simulink model "SupervisorFSM_TX"  (R2023b)
settings: Solver=FixedStepDiscrete  StartTime=0.0  StopTime=10.0  FixedStep=Ts_SupervisorFSM_TX  RelTol=1e-3  EnableMultiTasking=on
libraries: simulink x2
settings Model: DataDictionary=EmbeddedBoardDD.sldd  Creator=vvasco  LastModifiedBy=upattacini
settings SolverCC: AllowMultiTaskInputOutput=on  AlgebraicLoopSolver=TrustRegion  AutoInsertRateTranBlk=on  InsertRTBMode=Never (minimum delay)
settings DataIOCC: LimitDataPoints=on  SaveOutput=off  SignalLogging=off  DSMLogging=off  SaveTime=off  ReturnWorkspaceOutputs=off
settings OptimizationCC: DefaultParameterBehavior=Inlined  DefaultUnderspecifiedDataType=single  StrengthReduction=on  PassReuseOutputArgsAs=Individual arguments  ZeroExternalMemoryAtStartup=off  ZeroInternalMemoryAtStartup=off  OptimizeBlockOrder=speed  OptimizationPriority=Speed  OptimizationCustomize=off  MultiThreadedLoops=on  EfficientTunableParamExpr=on
settings DebuggingCC: ParameterPrecisionLossMsg=none  UnconnectedInputMsg=warning  UnconnectedOutputMsg=warning  UnconnectedLineMsg=warning  AllowSymbolicDim=off  SFUnexpectedBacktrackingDiag=warning  SFNoUnconditionalDefaultTransitionDiag=warning  SFExecutionAtInitializationDiag=none  ArithmeticOperatorsInVariantConditions=warning
settings HardwareCC: ProdBitPerPointer=32  ProdBitPerSizeT=32  ProdBitPerPtrDiffT=32  ProdLargestAtomicInteger=Long  ProdLargestAtomicFloat=Double  ProdWordSize=32  ProdHWDeviceType=ARM Compatible->ARM Cortex-M
settings ModelReferenceCC: UpdateModelReferenceTargets=Force  EnableRefExpFcnMdlSchedulingChecks=on  ModelReferenceNumInstancesAllowed=Single
settings SFSimCC: SimUseLocalCustomCode=off  MATLABDynamicMemAlloc=off  CustomCodeUndefinedFunction=UseInterfaceOnly
settings RTWCC: Description=Embedded Coder  SystemTargetFile=ert.tlc  GenCodeOnly=on  PackageGeneratedCodeAndArtifacts=on  PackageName=SupervisorFSM_TX  TemplateMakefile=ert_default_tmf  GenerateReport=on  RTWUseLocalCustomCode=off  LaunchReport=on  TargetLang=C++  GenerateCodeReplacementReport=on  DLArmComputeVersion=19.05
settings CodeAppCC: ForceParamTrailComments=on  IgnoreCustomStorageClasses=off  MaxIdLength=60  OperatorAnnotations=on  SimulinkDataObjDesc=on  SFDataObjDesc=on  InsertBlockDesc=on
settings ERTTargetCC: TargetLangStandard=C++03 (ISO)  CodeReplacementLibrary=ARM Cortex-M,iCubTech  GenerateSampleERTMain=on  SupportVariableSizeSignals=on  InlinedParameterPlacement=NonHierarchical  RootIOFormat=Structure reference  ERTCustomFileTemplate=example_file_process.tlc
settings ConfigComp: CovMetricSettings=dw  CovSaveCumulativeToWorkspaceVar=on  CovSaveSingleToWorkspaceVar=on  CovExternalEMLEnable=off

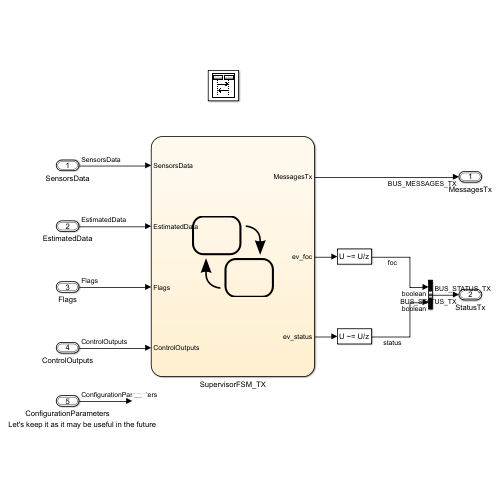
[thumbnail: Simulink's stored preview of the top-level diagram]
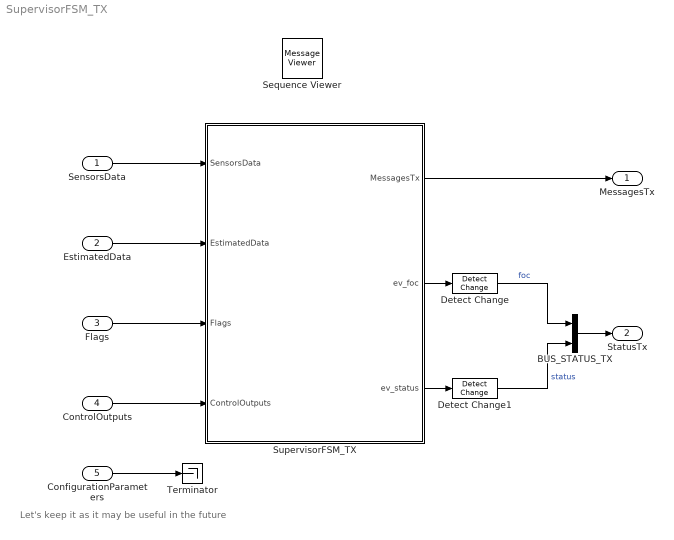
== system SupervisorFSM_TX ==
  note: Let's keep it as it may be useful in the future
  SensorsData : Inport  OutDataTypeStr=Bus: SensorsData  BusOutputAsStruct=on
  EstimatedData : Inport  Port=2  OutDataTypeStr=Bus: EstimatedData  BusOutputAsStruct=on
  Flags : Inport  Port=3  OutDataTypeStr=Bus: Flags  BusOutputAsStruct=on
  ControlOutputs : Inport  Port=4  OutDataTypeStr=Bus: ControlOutputs  BusOutputAsStruct=on
  ConfigurationParameters : Inport  Port=5  OutDataTypeStr=Bus: ConfigurationParameters  BusOutputAsStruct=on
  BUS_STATUS_TX : BusCreator  Inputs=2  OutDataTypeStr=Bus: BUS_STATUS_TX  NonVirtualBus=on
      settings: InheritFromInputs=off
  Detect Change : simulink/Logic and Bit Operations/Detect Change  vinit=false  OutDataTypeStr=boolean
  Detect Change1 : simulink/Logic and Bit Operations/Detect Change  vinit=false  OutDataTypeStr=boolean
  Sequence Viewer : MessageViewer  History=1000  SavedRootId=#
  SupervisorFSM_TX : Stateflow chart  TreatAsAtomicUnit=on
  Terminator : Terminator
  MessagesTx : Outport  OutDataTypeStr=Bus: BUS_MESSAGES_TX  BusOutputAsStruct=on
  StatusTx : Outport  Port=2  OutDataTypeStr=Bus: BUS_STATUS_TX  BusOutputAsStruct=on
  wires:
  SupervisorFSM_TX/1(MessagesTx) -> MessagesTx/1
  SensorsData/1 -> SupervisorFSM_TX/1(SensorsData)
  Flags/1 -> SupervisorFSM_TX/3(Flags)
  BUS_STATUS_TX/1 -> StatusTx/1
  EstimatedData/1 -> SupervisorFSM_TX/2(EstimatedData)
  ControlOutputs/1 -> SupervisorFSM_TX/4(ControlOutputs)
  SupervisorFSM_TX/2(ev_foc) -> Detect Change/1
  Detect Change/1 -> BUS_STATUS_TX/1  "foc"
  SupervisorFSM_TX/3(ev_status) -> Detect Change1/1
  Detect Change1/1 -> BUS_STATUS_TX/2  "status"
  ConfigurationParameters/1 -> Terminator/1

== stateflow chart SupervisorFSM_TX/SupervisorFSM_TX ==
  state MSG_FOC_HANDLER [parallel]
    settings: executionOrder=1
    state Home
    (default) -> MSG_FOC_HANDLER.Home
    MSG_FOC_HANDLER.Home -> MSG_FOC_HANDLER.Home : [Flags.enable_sending_msg_status]
        | {MessagesTx.foc.current = EstimatedData.Iq_filtered.current;
        | MessagesTx.foc.velocity = EstimatedData.jointvelocities.velocity;
        | MessagesTx.foc.position = SensorsData.jointpositions.position;
        | send(ev_foc);}
  state MSG_STATUS_HANDLER [parallel]
    settings: executionOrder=2
    state Home
    (default) -> MSG_STATUS_HANDLER.Home
    MSG_STATUS_HANDLER.Home -> MSG_STATUS_HANDLER.Home : [Flags.enable_sending_msg_status]
        | {MessagesTx.status.control_mode = convert(Flags.control_mode);
        | MessagesTx.status.pwm_fbk = ControlOutputs.Vq;
        | MessagesTx.status.flags.ExternalFaultAsserted = Flags.fault_button;
        | MessagesTx.status.flags.OverCurrentFailure = Flags.overcurrent;
        | send(ev_status);}
  data: mccontrolmode function_output Enum: MCControlModes size=1; controlmode function_input Enum: ControlModes size=1; MessagesTx output Bus: BUS_MESSAGES_TX; SensorsData input Bus: SensorsData; EstimatedData input Bus: EstimatedData; Flags input Bus: Flags; ControlOutputs input Bus: ControlOutputs
  events: ev_foc output EITHER_EDGE_EVENT; ev_status output EITHER_EDGE_EVENT
  function mccontrolmode = convert(controlmode):
    | function mccontrolmode = convert(controlmode)
    | 
    | if controlmode == ControlModes.Idle
    |     mccontrolmode = MCControlModes.Idle;
    | elseif controlmode == ControlModes.Current
    |     mccontrolmode = MCControlModes.Current;
    | elseif controlmode == ControlModes.Velocity
    |     mccontrolmode = MCControlModes.SpeedVoltage;
    | elseif controlmode == ControlModes.Voltage
    |     mccontrolmode = MCControlModes.OpenLoop;
    | elseif controlmode == ControlModes.HwFaultCM
    |     mccontrolmode = MCControlModes.HWFault;
    | else
    |     mccontrolmode = MCControlModes.Idle;
    | end
    | 
    | end
